simulink model "Parallel_n25_D2"  (R2012b)
settings: Solver=VariableStepDiscrete  StartTime=0.0  StopTime=TotalIterations  RelTol=1e-3
values from neighbouring files (symbols this model uses):
  bp = 12    [ConfigValidate.m]
  bpSNMemory = bp    (= 12)    [ConfigValidate.m]
  IterationsOrdering = 4000    [ConfigValidate.m]
  MaxCoordDistance = (abs(max(wx) - min(wx))+abs(max(wy) - min(wy)))^2    [ConfigValidate.m]
  N_limit = 0.01    [ConfigValidate.m]
  nBits = 9    [ConfigValidate.m]
  nBitsNSmemories = (ceil(log2(TotalIterations)))    [ConfigValidate.m]
  S_limit = 1    [ConfigValidate.m]
  SourceNodes = 2000    [ConfigValidate.m]
  ts = 1    [ConfigValidate.m]
  w1 = rand(1,Neurons)    [ConfigValidate.m]
  w2 = rand(1,Neurons)    [ConfigValidate.m]
  wx = zeros(1,Neurons)    [ConfigValidate.m]
  wy = zeros(1,Neurons)    [ConfigValidate.m]
  x1 = rand(SourceNodes,1)    [ConfigValidate.m]
  x2 = rand(SourceNodes,1)    [ConfigValidate.m]
libraries: xbsIndex_r4 x1652, dspsrcs4 x2, dspstat3 x2
(part 2 of 9)

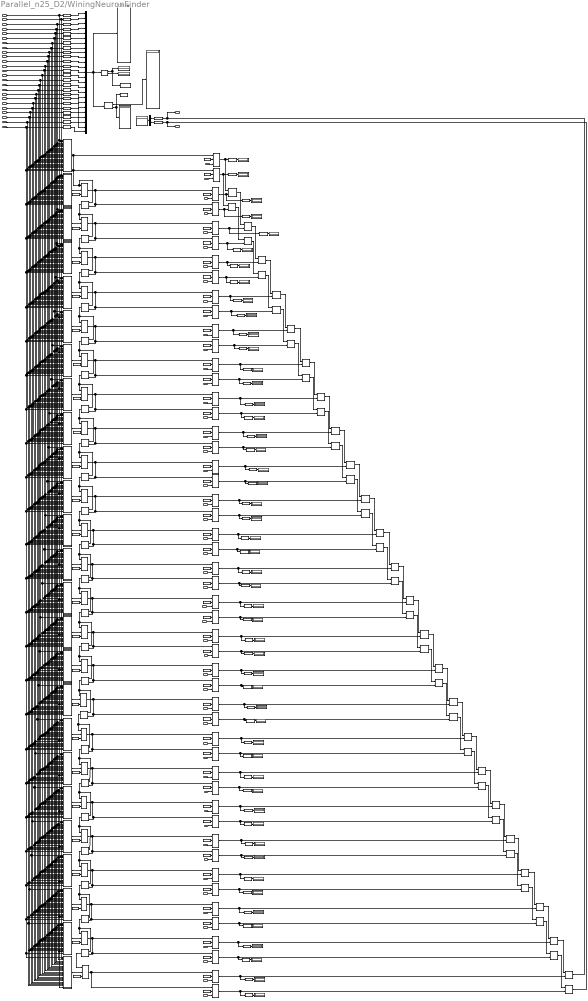
== system Parallel_n25_D2/WiningNeuronFinder ==
  dist_k1 : Inport
  dist_k2 : Inport  Port=2
  dist_k3 : Inport  Port=3
  dist_k4 : Inport  Port=4
  dist_k5 : Inport  Port=5
  dist_k6 : Inport  Port=6
  dist_k7 : Inport  Port=7
  dist_k8 : Inport  Port=8
  dist_k9 : Inport  Port=9
  dist_k10 : Inport  Port=10
  dist_k11 : Inport  Port=11
  dist_k12 : Inport  Port=12
  dist_k13 : Inport  Port=13
  dist_k14 : Inport  Port=14
  dist_k15 : Inport  Port=15
  dist_k16 : Inport  Port=16
  dist_k17 : Inport  Port=17
  dist_k18 : Inport  Port=18
  dist_k19 : Inport  Port=19
  dist_k20 : Inport  Port=20
  dist_k21 : Inport  Port=21
  dist_k22 : Inport  Port=22
  dist_k23 : Inport  Port=23
  dist_k24 : Inport  Port=24
  dist_k25 : Inport  Port=25
  wx_1 : Inport  Port=26
  wy_1 : Inport  Port=27
  wx_2 : Inport  Port=28
  wy_2 : Inport  Port=29
  wx_3 : Inport  Port=30
  wy_3 : Inport  Port=31
  wx_4 : Inport  Port=32
  wy_4 : Inport  Port=33
  wx_5 : Inport  Port=34
  wy_5 : Inport  Port=35
  wx_6 : Inport  Port=36
  wy_6 : Inport  Port=37
  wx_7 : Inport  Port=38
  wy_7 : Inport  Port=39
  wx_8 : Inport  Port=40
  wy_8 : Inport  Port=41
  wx_9 : Inport  Port=42
  wy_9 : Inport  Port=43
  wx_10 : Inport  Port=44
  wy_10 : Inport  Port=45
  wx_11 : Inport  Port=46
  wy_11 : Inport  Port=47
  wx_12 : Inport  Port=48
  wy_12 : Inport  Port=49
  wx_13 : Inport  Port=50
  wy_13 : Inport  Port=51
  wx_14 : Inport  Port=52
  wy_14 : Inport  Port=53
  wx_15 : Inport  Port=54
  wy_15 : Inport  Port=55
  wx_16 : Inport  Port=56
  wy_16 : Inport  Port=57
  wx_17 : Inport  Port=58
  wy_17 : Inport  Port=59
  wx_18 : Inport  Port=60
  wy_18 : Inport  Port=61
  wx_19 : Inport  Port=62
  wy_19 : Inport  Port=63
  wx_20 : Inport  Port=64
  wy_20 : Inport  Port=65
  wx_21 : Inport  Port=66
  wy_21 : Inport  Port=67
  wx_22 : Inport  Port=68
  wy_22 : Inport  Port=69
  wx_23 : Inport  Port=70
  wy_23 : Inport  Port=71
  wx_24 : Inport  Port=72
  wy_24 : Inport  Port=73
  wx_25 : Inport  Port=74
  wy_25 : Inport  Port=75
  Display{,1..55} (56 alike) : Display
  Gateway Out{,1..24,27..78} (77 alike) : xbsIndex_r4/Gateway Out  inherit_from_input=off  hdl_port=off  timing_constraint=None  locs_specified=off  LOCs={}  UseAsDAC=off  DACChannel='1'  block_type=gatewayout
  Logical{,1..22} (23 alike) : xbsIndex_r4/Logical  logical_function=OR  inputs=2  en=off  latency=0  precision=Full  arith_type=Unsigned  n_bits=16  bin_pt=0  align_bp=on  dbl_ovrd=off  block_type=logical
  LowerDist_n1 : Subsystem
  LowerDist_n10 : Subsystem
  LowerDist_n11 : Subsystem
  LowerDist_n12 : Subsystem
  LowerDist_n13 : Subsystem
  LowerDist_n14 : Subsystem
  LowerDist_n15 : Subsystem
  LowerDist_n16 : Subsystem
  LowerDist_n17 : Subsystem
  LowerDist_n18 : Subsystem
  LowerDist_n19 : Subsystem
  LowerDist_n2 : Subsystem
  LowerDist_n20 : Subsystem
  LowerDist_n21 : Subsystem
  LowerDist_n22 : Subsystem
  LowerDist_n23 : Subsystem
  LowerDist_n24 : Subsystem
  LowerDist_n25 : Subsystem
  LowerDist_n3 : Subsystem
  LowerDist_n4 : Subsystem
  LowerDist_n5 : Subsystem
  LowerDist_n6 : Subsystem
  LowerDist_n7 : Subsystem
  LowerDist_n8 : Subsystem
  LowerDist_n9 : Subsystem
  Minimum : dspstat3/Minimum  fcn=Value and Index  reset=None  InputProcessing=Columns as channels (frame based)  indexBase=One  operateOver=Each column  Dimension=1  colComp=on  operation=minimum  roiEnable=off  roiType=Rectangles  roiPortion=Entire ROI  roiOutput=Individual statistics for each ROI  roiFlag=off  roundingMode=Floor  overflowMode=off
  Mux : Mux  Inputs=25
  Mux2 : Mux  Inputs=2
  Sort : dspstat3/Sort  otype=Value and Index  dir=Ascending  sortAlg=Quick sort  accumDataTypeStr=Inherit: Same as product output  accumLastDataTypeStr=Inherit: Same as product output  roundingMode=Floor  overflowMode=off
  Sum_wxWinning_n{1..48} (48 alike) : xbsIndex_r4/AddSub  mode=Addition  use_carryin=off  use_carryout=off  en=off  latency=dAdd_CooperatingProcess  precision=User Defined  arith_type=Unsigned  n_bits=nbCoord  bin_pt=bpCoord  quantization=Truncate  overflow=Wrap  dbl_ovrd=off  use_behavioral_HDL=off  hw_selection=Fabric  pipelined=off  block_type=addsub
  To Workspace : ToWorkspace  VariableName=win_histH  SampleTime=ts
  To Workspace1 : ToWorkspace  VariableName=win_distH  SampleTime=ts
  wy_doMenor{,1..73} (74 alike) : xbsIndex_r4/Mux  inputs=2  en=off  latency=dMUX_CompetitiveProcess  precision=Full  arith_type=Unsigned  n_bits=16  bin_pt=14  quantization=Truncate  overflow=Wrap  dbl_ovrd=off  block_type=mux
  zero{,1..49} (50 alike) : xbsIndex_r4/Constant  const=0  gui_display_data_type=Fixed-point  arith_type=Unsigned  n_bits=nbCoord  bin_pt=bpCoord  preci_type=Single  exp_width=8  frac_width=24  explicit_period=on  period=ts  equ=P=C  opselect=C  inp2=PCIN>>17  opr=+  inp1=P  carry=CIN  dbl_ovrd=off  block_type=constant
  zero{50..73} (24 alike) : xbsIndex_r4/Constant  const=0  gui_display_data_type=Boolean  arith_type=Boolean  n_bits=nbCoord  bin_pt=bpCoord  preci_type=Single  exp_width=8  frac_width=24  explicit_period=on  period=ts  equ=P=C  opselect=C  inp2=PCIN>>17  opr=+  inp1=P  carry=CIN  dbl_ovrd=off  block_type=constant
  WinningNeuron_wx : Outport
  WinningNeuron_wy : Outport  Port=2
  wires:
  dist_k6/1 -> LowerDist_n25/6(In6), LowerDist_n24/6(In6), LowerDist_n23/6(In6), LowerDist_n22/6(In6), LowerDist_n21/6(In6), LowerDist_n20/6(In6), LowerDist_n19/6(In6), LowerDist_n18/6(In6), LowerDist_n17/6(In6), LowerDist_n16/6(In6), LowerDist_n15/6(In6), LowerDist_n14/6(In6), LowerDist_n13/6(In6), LowerDist_n12/6(In6), LowerDist_n11/6(In6), LowerDist_n10/6(In6), LowerDist_n9/6(In6), LowerDist_n8/6(In6), LowerDist_n7/6(In6), LowerDist_n6/1(In1), LowerDist_n5/6(In6), LowerDist_n4/6(In6), LowerDist_n3/6(In6), LowerDist_n2/6(In6), LowerDist_n1/6(In6), Gateway Out5/1
  wy_1/1 -> wy_doMenor1/3
  wx_2/1 -> wy_doMenor2/3
  wy_2/1 -> wy_doMenor3/3
  wx_3/1 -> wy_doMenor4/3
  wy_3/1 -> wy_doMenor5/3
  wx_4/1 -> wy_doMenor6/3
  wy_4/1 -> wy_doMenor7/3
  wx_5/1 -> wy_doMenor8/3
  wy_5/1 -> wy_doMenor9/3
  wx_6/1 -> wy_doMenor10/3
  wy_6/1 -> wy_doMenor11/3
  wx_7/1 -> wy_doMenor12/3
  wy_7/1 -> wy_doMenor13/3
  wx_8/1 -> wy_doMenor14/3
  wy_8/1 -> wy_doMenor15/3
  wx_9/1 -> wy_doMenor16/3
  wy_9/1 -> wy_doMenor17/3
  wx_10/1 -> wy_doMenor18/3
  wy_10/1 -> wy_doMenor19/3
  wx_11/1 -> wy_doMenor20/3
  wy_11/1 -> wy_doMenor21/3
  wx_12/1 -> wy_doMenor22/3
  wy_12/1 -> wy_doMenor23/3
  wx_13/1 -> wy_doMenor24/3
  wy_13/1 -> wy_doMenor25/3
  wx_14/1 -> wy_doMenor26/3
  wy_14/1 -> wy_doMenor27/3
  wx_15/1 -> wy_doMenor28/3
  wy_15/1 -> wy_doMenor29/3
  wx_16/1 -> wy_doMenor30/3
  wy_16/1 -> wy_doMenor31/3
  wx_17/1 -> wy_doMenor32/3
  wy_17/1 -> wy_doMenor33/3
  wx_18/1 -> wy_doMenor34/3
  wy_18/1 -> wy_doMenor35/3
  wx_19/1 -> wy_doMenor36/3
  wy_19/1 -> wy_doMenor37/3
  wx_20/1 -> wy_doMenor38/3
  wy_20/1 -> wy_doMenor39/3
  wx_21/1 -> wy_doMenor40/3
  wy_21/1 -> wy_doMenor41/3
  wx_22/1 -> wy_doMenor42/3
  wy_22/1 -> wy_doMenor43/3
  wx_23/1 -> wy_doMenor44/3
  wy_23/1 -> wy_doMenor45/3
  wx_24/1 -> wy_doMenor46/3
  wy_24/1 -> wy_doMenor47/3
  wx_25/1 -> wy_doMenor48/3
  wy_25/1 -> wy_doMenor49/3
  wx_1/1 -> wy_doMenor/3
  Gateway Out6/1 -> Mux/7
  Gateway Out5/1 -> Mux/6
  Gateway Out7/1 -> Mux/8
  Gateway Out4/1 -> Mux/5
  Gateway Out8/1 -> Mux/9
  Gateway Out1/1 -> Mux/2
  Gateway Out3/1 -> Mux/4
  Gateway Out2/1 -> Mux/3
  Gateway Out10/1 -> Mux/11
  Gateway Out11/1 -> Mux/12
  Gateway Out9/1 -> Mux/10
  Gateway Out/1 -> Mux/1
  Gateway Out12/1 -> Mux/13
  Gateway Out22/1 -> Mux/17
  Gateway Out13/1 -> Mux/14
  Gateway Out14/1 -> Mux/15
  Gateway Out15/1 -> Mux/16
  Gateway Out23/1 -> Mux/18
  Gateway Out16/1 -> Mux/20
  Gateway Out17/1 -> Mux/21
  Gateway Out24/1 -> Mux/19
  Gateway Out18/1 -> Mux/22
  Gateway Out20/1 -> Mux/24
  Gateway Out21/1 -> Mux/25
  Gateway Out19/1 -> Mux/23
  dist_k3/1 -> LowerDist_n1/3(In3), LowerDist_n25/3(In3), LowerDist_n24/3(In3), LowerDist_n23/3(In3), LowerDist_n22/3(In3), LowerDist_n21/3(In3), LowerDist_n20/3(In3), LowerDist_n19/3(In3), LowerDist_n18/3(In3), LowerDist_n17/3(In3), LowerDist_n16/3(In3), LowerDist_n15/3(In3), LowerDist_n14/3(In3), LowerDist_n13/3(In3), LowerDist_n12/3(In3), LowerDist_n11/3(In3), LowerDist_n10/3(In3), LowerDist_n9/3(In3), LowerDist_n8/3(In3), LowerDist_n7/3(In3), LowerDist_n6/3(In3), LowerDist_n5/3(In3), LowerDist_n4/3(In3), LowerDist_n3/1(In1), LowerDist_n2/3(In3), Gateway Out2/1
  dist_k25/1 -> LowerDist_n6/25(In25), LowerDist_n12/25(In25), LowerDist_n15/25(In25), LowerDist_n21/25(In25), LowerDist_n25/1(In1), LowerDist_n24/25(In25), LowerDist_n23/25(In25), LowerDist_n22/25(In25), LowerDist_n20/25(In25), LowerDist_n19/25(In25), LowerDist_n18/25(In25), LowerDist_n17/25(In25), LowerDist_n16/25(In25), LowerDist_n14/25(In25), LowerDist_n13/25(In25), LowerDist_n11/25(In25), LowerDist_n10/25(In25), LowerDist_n9/25(In25), LowerDist_n8/25(In25), LowerDist_n7/25(In25), LowerDist_n5/25(In25), LowerDist_n4/25(In25), LowerDist_n3/25(In25), LowerDist_n2/25(In25), LowerDist_n1/25(In25), Gateway Out21/1
  dist_k15/1 -> LowerDist_n20/15(In15), LowerDist_n25/15(In15), LowerDist_n24/15(In15), LowerDist_n23/15(In15), LowerDist_n22/15(In15), LowerDist_n21/15(In15), LowerDist_n19/15(In15), LowerDist_n18/15(In15), LowerDist_n17/15(In15), LowerDist_n16/15(In15), LowerDist_n15/1(In1), LowerDist_n14/15(In15), LowerDist_n13/15(In15), LowerDist_n12/15(In15), LowerDist_n11/15(In15), LowerDist_n10/15(In15), LowerDist_n9/15(In15), LowerDist_n8/15(In15), LowerDist_n7/15(In15), LowerDist_n6/15(In15), LowerDist_n5/15(In15), LowerDist_n4/15(In15), LowerDist_n3/15(In15), LowerDist_n2/15(In15), LowerDist_n1/15(In15), Gateway Out14/1
  dist_k2/1 -> LowerDist_n25/2(In2), LowerDist_n24/2(In2), LowerDist_n23/2(In2), LowerDist_n22/2(In2), LowerDist_n21/2(In2), LowerDist_n20/2(In2), LowerDist_n19/2(In2), LowerDist_n18/2(In2), LowerDist_n17/2(In2), LowerDist_n16/2(In2), LowerDist_n15/2(In2), LowerDist_n14/2(In2), LowerDist_n13/2(In2), LowerDist_n12/2(In2), LowerDist_n11/2(In2), LowerDist_n10/2(In2), LowerDist_n9/2(In2), LowerDist_n8/2(In2), LowerDist_n7/2(In2), LowerDist_n6/2(In2), LowerDist_n5/2(In2), LowerDist_n4/2(In2), LowerDist_n3/2(In2), LowerDist_n2/1(In1), LowerDist_n1/2(In2), Gateway Out1/1
  dist_k4/1 -> LowerDist_n2/4(In4), LowerDist_n8/4(In4), LowerDist_n25/4(In4), LowerDist_n24/4(In4), LowerDist_n23/4(In4), LowerDist_n22/4(In4), LowerDist_n21/4(In4), LowerDist_n20/4(In4), LowerDist_n19/4(In4), LowerDist_n18/4(In4), LowerDist_n17/4(In4), LowerDist_n16/4(In4), LowerDist_n15/4(In4), LowerDist_n14/4(In4), LowerDist_n13/4(In4), LowerDist_n12/4(In4), LowerDist_n11/4(In4), LowerDist_n10/4(In4), LowerDist_n9/4(In4), LowerDist_n7/4(In4), LowerDist_n6/4(In4), LowerDist_n5/4(In4), LowerDist_n4/1(In1), LowerDist_n3/4(In4), LowerDist_n1/4(In4), Gateway Out3/1
  dist_k7/1 -> LowerDist_n25/7(In7), LowerDist_n24/7(In7), LowerDist_n23/7(In7), LowerDist_n22/7(In7), LowerDist_n21/7(In7), LowerDist_n20/7(In7), LowerDist_n19/7(In7), LowerDist_n18/7(In7), LowerDist_n17/7(In7), LowerDist_n16/7(In7), LowerDist_n15/7(In7), LowerDist_n14/7(In7), LowerDist_n13/7(In7), LowerDist_n12/7(In7), LowerDist_n11/7(In7), LowerDist_n10/7(In7), LowerDist_n9/7(In7), LowerDist_n8/7(In7), LowerDist_n7/1(In1), LowerDist_n6/7(In7), LowerDist_n5/7(In7), LowerDist_n4/7(In7), LowerDist_n3/7(In7), LowerDist_n2/7(In7), LowerDist_n1/7(In7), Gateway Out6/1
  dist_k8/1 -> LowerDist_n8/1(In1), LowerDist_n25/8(In8), LowerDist_n24/8(In8), LowerDist_n23/8(In8), LowerDist_n22/8(In8), LowerDist_n21/8(In8), LowerDist_n20/8(In8), LowerDist_n19/8(In8), LowerDist_n18/8(In8), LowerDist_n17/8(In8), LowerDist_n16/8(In8), LowerDist_n15/8(In8), LowerDist_n14/8(In8), LowerDist_n13/8(In8), LowerDist_n12/8(In8), LowerDist_n11/8(In8), LowerDist_n10/8(In8), LowerDist_n9/8(In8), LowerDist_n7/8(In8), LowerDist_n6/8(In8), LowerDist_n5/8(In8), LowerDist_n4/8(In8), LowerDist_n3/8(In8), LowerDist_n2/8(In8), LowerDist_n1/8(In8), Gateway Out7/1
  dist_k9/1 -> LowerDist_n20/9(In9), LowerDist_n22/9(In9), LowerDist_n24/9(In9), LowerDist_n25/9(In9), LowerDist_n23/9(In9), LowerDist_n21/9(In9), LowerDist_n19/9(In9), LowerDist_n18/9(In9), LowerDist_n17/9(In9), LowerDist_n16/9(In9), LowerDist_n15/9(In9), LowerDist_n14/9(In9), LowerDist_n13/9(In9), LowerDist_n12/9(In9), LowerDist_n11/9(In9), LowerDist_n10/9(In9), LowerDist_n9/1(In1), LowerDist_n8/9(In9), LowerDist_n7/9(In9), LowerDist_n6/9(In9), LowerDist_n5/9(In9), LowerDist_n4/9(In9), LowerDist_n3/9(In9), LowerDist_n2/9(In9), LowerDist_n1/9(In9), Gateway Out8/1
  dist_k10/1 -> LowerDist_n9/10(In10), LowerDist_n25/10(In10), LowerDist_n24/10(In10), LowerDist_n23/10(In10), LowerDist_n22/10(In10), LowerDist_n21/10(In10), LowerDist_n20/10(In10), LowerDist_n19/10(In10), LowerDist_n18/10(In10), LowerDist_n17/10(In10), LowerDist_n16/10(In10), LowerDist_n15/10(In10), LowerDist_n14/10(In10), LowerDist_n13/10(In10), LowerDist_n12/10(In10), LowerDist_n11/10(In10), LowerDist_n10/1(In1), LowerDist_n8/10(In10), LowerDist_n7/10(In10), LowerDist_n6/10(In10), LowerDist_n5/10(In10), LowerDist_n4/10(In10), LowerDist_n3/10(In10), LowerDist_n2/10(In10), LowerDist_n1/10(In10), Gateway Out9/1
  dist_k11/1 -> LowerDist_n11/1(In1), LowerDist_n25/11(In11), LowerDist_n24/11(In11), LowerDist_n23/11(In11), LowerDist_n22/11(In11), LowerDist_n21/11(In11), LowerDist_n20/11(In11), LowerDist_n19/11(In11), LowerDist_n18/11(In11), LowerDist_n17/11(In11), LowerDist_n16/11(In11), LowerDist_n15/11(In11), LowerDist_n14/11(In11), LowerDist_n13/11(In11), LowerDist_n12/11(In11), LowerDist_n10/11(In11), LowerDist_n9/11(In11), LowerDist_n8/11(In11), LowerDist_n7/11(In11), LowerDist_n6/11(In11), LowerDist_n5/11(In11), LowerDist_n4/11(In11), LowerDist_n3/11(In11), LowerDist_n2/11(In11), LowerDist_n1/11(In11), Gateway Out10/1
  dist_k12/1 -> LowerDist_n11/12(In12), LowerDist_n23/12(In12), LowerDist_n25/12(In12), LowerDist_n24/12(In12), LowerDist_n22/12(In12), LowerDist_n21/12(In12), LowerDist_n20/12(In12), LowerDist_n19/12(In12), LowerDist_n18/12(In12), LowerDist_n17/12(In12), LowerDist_n16/12(In12), LowerDist_n15/12(In12), LowerDist_n14/12(In12), LowerDist_n13/12(In12), LowerDist_n12/1(In1), LowerDist_n10/12(In12), LowerDist_n9/12(In12), LowerDist_n8/12(In12), LowerDist_n7/12(In12), LowerDist_n6/12(In12), LowerDist_n5/12(In12), LowerDist_n4/12(In12), LowerDist_n3/12(In12), LowerDist_n2/12(In12), LowerDist_n1/12(In12), Gateway Out11/1
  dist_k13/1 -> LowerDist_n12/13(In13), LowerDist_n25/13(In13), LowerDist_n24/13(In13), LowerDist_n23/13(In13), LowerDist_n22/13(In13), LowerDist_n21/13(In13), LowerDist_n20/13(In13), LowerDist_n19/13(In13), LowerDist_n18/13(In13), LowerDist_n17/13(In13), LowerDist_n16/13(In13), LowerDist_n15/13(In13), LowerDist_n14/13(In13), LowerDist_n13/1(In1), LowerDist_n11/13(In13), LowerDist_n10/13(In13), LowerDist_n9/13(In13), LowerDist_n8/13(In13), LowerDist_n7/13(In13), LowerDist_n6/13(In13), LowerDist_n5/13(In13), LowerDist_n4/13(In13), LowerDist_n3/13(In13), LowerDist_n2/13(In13), LowerDist_n1/13(In13), Gateway Out12/1
  dist_k14/1 -> LowerDist_n14/1(In1), LowerDist_n21/14(In14), LowerDist_n25/14(In14), LowerDist_n24/14(In14), LowerDist_n23/14(In14), LowerDist_n22/14(In14), LowerDist_n20/14(In14), LowerDist_n19/14(In14), LowerDist_n18/14(In14), LowerDist_n17/14(In14), LowerDist_n16/14(In14), LowerDist_n15/14(In14), LowerDist_n13/14(In14), LowerDist_n12/14(In14), LowerDist_n11/14(In14), LowerDist_n10/14(In14), LowerDist_n9/14(In14), LowerDist_n8/14(In14), LowerDist_n7/14(In14), LowerDist_n6/14(In14), LowerDist_n5/14(In14), LowerDist_n4/14(In14), LowerDist_n3/14(In14), LowerDist_n2/14(In14), LowerDist_n1/14(In14), Gateway Out13/1
  dist_k16/1 -> LowerDist_n1/16(In16), LowerDist_n10/16(In16), LowerDist_n15/16(In16), LowerDist_n25/16(In16), LowerDist_n24/16(In16), LowerDist_n23/16(In16), LowerDist_n22/16(In16), LowerDist_n21/16(In16), LowerDist_n20/16(In16), LowerDist_n19/16(In16), LowerDist_n18/16(In16), LowerDist_n17/16(In16), LowerDist_n16/1(In1), LowerDist_n14/16(In16), LowerDist_n13/16(In16), LowerDist_n12/16(In16), LowerDist_n11/16(In16), LowerDist_n9/16(In16), LowerDist_n8/16(In16), LowerDist_n7/16(In16), LowerDist_n6/16(In16), LowerDist_n5/16(In16), LowerDist_n4/16(In16), LowerDist_n3/16(In16), LowerDist_n2/16(In16), Gateway Out15/1
  dist_k17/1 -> LowerDist_n1/17(In17), LowerDist_n13/17(In17), LowerDist_n25/17(In17), LowerDist_n24/17(In17), LowerDist_n23/17(In17), LowerDist_n22/17(In17), LowerDist_n21/17(In17), LowerDist_n20/17(In17), LowerDist_n19/17(In17), LowerDist_n18/17(In17), LowerDist_n17/1(In1), LowerDist_n16/17(In17), LowerDist_n15/17(In17), LowerDist_n14/17(In17), LowerDist_n12/17(In17), LowerDist_n11/17(In17), LowerDist_n10/17(In17), LowerDist_n9/17(In17), LowerDist_n8/17(In17), LowerDist_n7/17(In17), LowerDist_n6/17(In17), LowerDist_n5/17(In17), LowerDist_n4/17(In17), LowerDist_n3/17(In17), LowerDist_n2/17(In17), Gateway Out22/1
  dist_k18/1 -> LowerDist_n17/18(In18), LowerDist_n25/18(In18), LowerDist_n24/18(In18), LowerDist_n23/18(In18), LowerDist_n22/18(In18), LowerDist_n21/18(In18), LowerDist_n20/18(In18), LowerDist_n19/18(In18), LowerDist_n18/1(In1), LowerDist_n16/18(In18), LowerDist_n15/18(In18), LowerDist_n14/18(In18), LowerDist_n13/18(In18), LowerDist_n12/18(In18), LowerDist_n11/18(In18), LowerDist_n10/18(In18), LowerDist_n9/18(In18), LowerDist_n8/18(In18), LowerDist_n7/18(In18), LowerDist_n6/18(In18), LowerDist_n5/18(In18), LowerDist_n4/18(In18), LowerDist_n3/18(In18), LowerDist_n2/18(In18), LowerDist_n1/18(In18), Gateway Out23/1
  dist_k19/1 -> LowerDist_n25/19(In19), LowerDist_n24/19(In19), LowerDist_n23/19(In19), LowerDist_n22/19(In19), LowerDist_n21/19(In19), LowerDist_n20/19(In19), LowerDist_n19/1(In1), LowerDist_n18/19(In19), LowerDist_n17/19(In19), LowerDist_n16/19(In19), LowerDist_n15/19(In19), LowerDist_n14/19(In19), LowerDist_n13/19(In19), LowerDist_n12/19(In19), LowerDist_n11/19(In19), LowerDist_n10/19(In19), LowerDist_n9/19(In19), LowerDist_n8/19(In19), LowerDist_n7/19(In19), LowerDist_n6/19(In19), LowerDist_n5/19(In19), LowerDist_n4/19(In19), LowerDist_n3/19(In19), LowerDist_n2/19(In19), LowerDist_n1/19(In19), Gateway Out24/1
  dist_k21/1 -> LowerDist_n9/21(In21), LowerDist_n25/21(In21), LowerDist_n24/21(In21), LowerDist_n23/21(In21), LowerDist_n22/21(In21), LowerDist_n21/1(In1), LowerDist_n20/21(In21), LowerDist_n19/21(In21), LowerDist_n18/21(In21), LowerDist_n17/21(In21), LowerDist_n16/21(In21), LowerDist_n15/21(In21), LowerDist_n14/21(In21), LowerDist_n13/21(In21), LowerDist_n12/21(In21), LowerDist_n11/21(In21), LowerDist_n10/21(In21), LowerDist_n8/21(In21), LowerDist_n7/21(In21), LowerDist_n6/21(In21), LowerDist_n5/21(In21), LowerDist_n4/21(In21), LowerDist_n3/21(In21), LowerDist_n2/21(In21), LowerDist_n1/21(In21), Gateway Out17/1
  dist_k22/1 -> LowerDist_n7/22(In22), LowerDist_n25/22(In22), LowerDist_n24/22(In22), LowerDist_n23/22(In22), LowerDist_n22/1(In1), LowerDist_n21/22(In22), LowerDist_n20/22(In22), LowerDist_n19/22(In22), LowerDist_n18/22(In22), LowerDist_n17/22(In22), LowerDist_n16/22(In22), LowerDist_n15/22(In22), LowerDist_n14/22(In22), LowerDist_n13/22(In22), LowerDist_n12/22(In22), LowerDist_n11/22(In22), LowerDist_n10/22(In22), LowerDist_n9/22(In22), LowerDist_n8/22(In22), LowerDist_n6/22(In22), LowerDist_n5/22(In22), LowerDist_n4/22(In22), LowerDist_n3/22(In22), LowerDist_n2/22(In22), LowerDist_n1/22(In22), Gateway Out18/1
  dist_k23/1 -> LowerDist_n25/23(In23), LowerDist_n24/23(In23), LowerDist_n23/1(In1), LowerDist_n22/23(In23), LowerDist_n21/23(In23), LowerDist_n20/23(In23), LowerDist_n19/23(In23), LowerDist_n18/23(In23), LowerDist_n17/23(In23), LowerDist_n16/23(In23), LowerDist_n15/23(In23), LowerDist_n14/23(In23), LowerDist_n13/23(In23), LowerDist_n12/23(In23), LowerDist_n11/23(In23), LowerDist_n10/23(In23), LowerDist_n9/23(In23), LowerDist_n8/23(In23), LowerDist_n7/23(In23), LowerDist_n6/23(In23), LowerDist_n5/23(In23), LowerDist_n4/23(In23), LowerDist_n3/23(In23), LowerDist_n2/23(In23), LowerDist_n1/23(In23), Gateway Out19/1
  dist_k24/1 -> LowerDist_n25/24(In24), LowerDist_n24/1(In1), LowerDist_n23/24(In24), LowerDist_n22/24(In24), LowerDist_n21/24(In24), LowerDist_n20/24(In24), LowerDist_n19/24(In24), LowerDist_n18/24(In24), LowerDist_n17/24(In24), LowerDist_n16/24(In24), LowerDist_n15/24(In24), LowerDist_n14/24(In24), LowerDist_n13/24(In24), LowerDist_n12/24(In24), LowerDist_n11/24(In24), LowerDist_n10/24(In24), LowerDist_n9/24(In24), LowerDist_n8/24(In24), LowerDist_n7/24(In24), LowerDist_n6/24(In24), LowerDist_n5/24(In24), LowerDist_n4/24(In24), LowerDist_n3/24(In24), LowerDist_n2/24(In24), LowerDist_n1/24(In24), Gateway Out20/1
  dist_k1/1 -> LowerDist_n1/1(In1), LowerDist_n4/4(In4), LowerDist_n25/25(In25), LowerDist_n24/24(In24), LowerDist_n23/23(In23), LowerDist_n22/22(In22), LowerDist_n21/21(In21), LowerDist_n20/20(In20), LowerDist_n19/19(In19), LowerDist_n18/18(In18), LowerDist_n17/17(In17), LowerDist_n16/16(In16), LowerDist_n15/15(In15), LowerDist_n14/14(In14), LowerDist_n13/13(In13), LowerDist_n12/12(In12), LowerDist_n11/11(In11), LowerDist_n10/10(In10), LowerDist_n9/9(In9), LowerDist_n8/8(In8), LowerDist_n7/7(In7), LowerDist_n6/6(In6), LowerDist_n5/5(In5), LowerDist_n3/3(In3), LowerDist_n2/2(In2), Gateway Out/1
  dist_k20/1 -> LowerDist_n14/20(In20), LowerDist_n25/20(In20), LowerDist_n24/20(In20), LowerDist_n23/20(In20), LowerDist_n22/20(In20), LowerDist_n21/20(In20), LowerDist_n20/1(In1), LowerDist_n19/20(In20), LowerDist_n18/20(In20), LowerDist_n17/20(In20), LowerDist_n16/20(In20), LowerDist_n15/20(In20), LowerDist_n13/20(In20), LowerDist_n12/20(In20), LowerDist_n11/20(In20), LowerDist_n10/20(In20), LowerDist_n9/20(In20), LowerDist_n8/20(In20), LowerDist_n7/20(In20), LowerDist_n6/20(In20), LowerDist_n5/20(In20), LowerDist_n4/20(In20), LowerDist_n3/20(In20), LowerDist_n2/20(In20), LowerDist_n1/20(In20), Gateway Out16/1
  zero/1 -> wy_doMenor/2
  zero1/1 -> wy_doMenor1/2
  zero2/1 -> wy_doMenor2/2
  zero3/1 -> wy_doMenor3/2
  zero4/1 -> wy_doMenor4/2
  zero5/1 -> wy_doMenor5/2
  zero6/1 -> wy_doMenor6/2
  zero7/1 -> wy_doMenor7/2
  zero8/1 -> wy_doMenor8/2
  zero9/1 -> wy_doMenor9/2
  zero10/1 -> wy_doMenor10/2
  zero11/1 -> wy_doMenor11/2
  zero12/1 -> wy_doMenor12/2
  zero13/1 -> wy_doMenor13/2
  zero14/1 -> wy_doMenor14/2
  zero15/1 -> wy_doMenor15/2
  zero16/1 -> wy_doMenor16/2
  zero17/1 -> wy_doMenor17/2
  zero18/1 -> wy_doMenor18/2
  zero19/1 -> wy_doMenor19/2
  zero20/1 -> wy_doMenor20/2
  zero21/1 -> wy_doMenor21/2
  zero22/1 -> wy_doMenor22/2
  zero23/1 -> wy_doMenor23/2
  zero24/1 -> wy_doMenor24/2
  zero25/1 -> wy_doMenor25/2
  zero26/1 -> wy_doMenor26/2
  zero27/1 -> wy_doMenor27/2
  zero28/1 -> wy_doMenor28/2
  zero29/1 -> wy_doMenor29/2
  zero30/1 -> wy_doMenor30/2
  zero31/1 -> wy_doMenor31/2
  zero32/1 -> wy_doMenor32/2
  zero33/1 -> wy_doMenor33/2
  zero34/1 -> wy_doMenor34/2
  zero35/1 -> wy_doMenor35/2
  zero36/1 -> wy_doMenor36/2
  zero37/1 -> wy_doMenor37/2
  zero38/1 -> wy_doMenor38/2
  zero39/1 -> wy_doMenor39/2
  zero40/1 -> wy_doMenor40/2
  zero41/1 -> wy_doMenor41/2
  zero42/1 -> wy_doMenor42/2
  zero43/1 -> wy_doMenor43/2
  zero44/1 -> wy_doMenor44/2
  zero45/1 -> wy_doMenor45/2
  zero46/1 -> wy_doMenor46/2
  zero47/1 -> wy_doMenor47/2
  zero48/1 -> wy_doMenor48/2
  zero49/1 -> wy_doMenor49/2
  wy_doMenor/1 -> Gateway Out29/1, Sum_wxWinning_n1/1
  wy_doMenor2/1 -> Gateway Out31/1, Sum_wxWinning_n1/2
  wy_doMenor1/1 -> Gateway Out30/1, Sum_wxWinning_n2/1
  wy_doMenor3/1 -> Gateway Out32/1, Sum_wxWinning_n2/2
  Sum_wxWinning_n1/1 -> Sum_wxWinning_n3/1
  Sum_wxWinning_n2/1 -> Sum_wxWinning_n4/1
  wy_doMenor4/1 -> Gateway Out34/1, Sum_wxWinning_n3/2
  wy_doMenor5/1 -> Gateway Out33/1, Sum_wxWinning_n4/2
  Sum_wxWinning_n3/1 -> Sum_wxWinning_n5/1
  Sum_wxWinning_n4/1 -> Sum_wxWinning_n6/1
  wy_doMenor6/1 -> Gateway Out35/1, Sum_wxWinning_n5/2
  wy_doMenor7/1 -> Gateway Out36/1, Sum_wxWinning_n6/2
  Sum_wxWinning_n5/1 -> Sum_wxWinning_n7/1
  Sum_wxWinning_n6/1 -> Sum_wxWinning_n8/1
  wy_doMenor9/1 -> Gateway Out38/1, Sum_wxWinning_n8/2
  Sum_wxWinning_n7/1 -> Sum_wxWinning_n9/1
  Sum_wxWinning_n8/1 -> Sum_wxWinning_n10/1
  wy_doMenor10/1 -> Gateway Out39/1, Sum_wxWinning_n9/2
  wy_doMenor11/1 -> Gateway Out40/1, Sum_wxWinning_n10/2
  Sum_wxWinning_n9/1 -> Sum_wxWinning_n12/1
  Sum_wxWinning_n10/1 -> Sum_wxWinning_n11/1
  wy_doMenor12/1 -> Gateway Out41/1, Sum_wxWinning_n12/2
  wy_doMenor13/1 -> Gateway Out42/1, Sum_wxWinning_n11/2
  Sum_wxWinning_n12/1 -> Sum_wxWinning_n14/1
  Sum_wxWinning_n11/1 -> Sum_wxWinning_n13/1
  wy_doMenor14/1 -> Gateway Out43/1, Sum_wxWinning_n14/2
  wy_doMenor15/1 -> Gateway Out44/1, Sum_wxWinning_n13/2
  Sum_wxWinning_n14/1 -> Sum_wxWinning_n16/1
  Sum_wxWinning_n13/1 -> Sum_wxWinning_n15/1
  wy_doMenor16/1 -> Gateway Out45/1, Sum_wxWinning_n16/2
  wy_doMenor17/1 -> Gateway Out46/1, Sum_wxWinning_n15/2
  Sum_wxWinning_n16/1 -> Sum_wxWinning_n18/1
  Sum_wxWinning_n15/1 -> Sum_wxWinning_n17/1
  wy_doMenor18/1 -> Gateway Out47/1, Sum_wxWinning_n18/2
  wy_doMenor19/1 -> Gateway Out48/1, Sum_wxWinning_n17/2
  Sum_wxWinning_n18/1 -> Sum_wxWinning_n20/1
  Sum_wxWinning_n17/1 -> Sum_wxWinning_n19/1
  wy_doMenor20/1 -> Gateway Out49/1, Sum_wxWinning_n20/2
  wy_doMenor21/1 -> Gateway Out50/1, Sum_wxWinning_n19/2
  Sum_wxWinning_n20/1 -> Sum_wxWinning_n22/1
  Sum_wxWinning_n19/1 -> Sum_wxWinning_n21/1
  wy_doMenor22/1 -> Gateway Out51/1, Sum_wxWinning_n22/2
  Sum_wxWinning_n22/1 -> Sum_wxWinning_n24/1
  Sum_wxWinning_n21/1 -> Sum_wxWinning_n23/1
  wy_doMenor24/1 -> Gateway Out53/1, Sum_wxWinning_n24/2
  wy_doMenor25/1 -> Gateway Out54/1, Sum_wxWinning_n23/2
  Sum_wxWinning_n24/1 -> Sum_wxWinning_n26/1
  Sum_wxWinning_n23/1 -> Sum_wxWinning_n25/1
  wy_doMenor26/1 -> Gateway Out55/1, Sum_wxWinning_n26/2
  wy_doMenor27/1 -> Gateway Out56/1, Sum_wxWinning_n25/2
  Sum_wxWinning_n26/1 -> Sum_wxWinning_n28/1
  Sum_wxWinning_n25/1 -> Sum_wxWinning_n27/1
  wy_doMenor28/1 -> Gateway Out57/1, Sum_wxWinning_n28/2
  wy_doMenor29/1 -> Gateway Out58/1, Sum_wxWinning_n27/2
  Sum_wxWinning_n28/1 -> Sum_wxWinning_n30/1
  Sum_wxWinning_n27/1 -> Sum_wxWinning_n29/1
  wy_doMenor30/1 -> Gateway Out59/1, Sum_wxWinning_n30/2
  wy_doMenor31/1 -> Gateway Out60/1, Sum_wxWinning_n29/2
  Sum_wxWinning_n30/1 -> Sum_wxWinning_n32/1
  Sum_wxWinning_n29/1 -> Sum_wxWinning_n31/1
  wy_doMenor32/1 -> Gateway Out61/1, Sum_wxWinning_n32/2
  wy_doMenor33/1 -> Gateway Out62/1, Sum_wxWinning_n31/2
  Sum_wxWinning_n32/1 -> Sum_wxWinning_n34/1
  Sum_wxWinning_n31/1 -> Sum_wxWinning_n33/1
  wy_doMenor34/1 -> Gateway Out63/1, Sum_wxWinning_n34/2
  wy_doMenor35/1 -> Gateway Out64/1, Sum_wxWinning_n33/2
  Sum_wxWinning_n34/1 -> Sum_wxWinning_n36/1
  Sum_wxWinning_n33/1 -> Sum_wxWinning_n35/1
  wy_doMenor36/1 -> Gateway Out65/1, Sum_wxWinning_n36/2
  wy_doMenor37/1 -> Gateway Out66/1, Sum_wxWinning_n35/2
  Sum_wxWinning_n36/1 -> Sum_wxWinning_n38/1
  Sum_wxWinning_n35/1 -> Sum_wxWinning_n37/1
  wy_doMenor38/1 -> Gateway Out67/1, Sum_wxWinning_n38/2
  wy_doMenor39/1 -> Gateway Out68/1, Sum_wxWinning_n37/2
  Sum_wxWinning_n38/1 -> Sum_wxWinning_n40/1
  Sum_wxWinning_n37/1 -> Sum_wxWinning_n39/1
  wy_doMenor40/1 -> Gateway Out69/1, Sum_wxWinning_n40/2
  wy_doMenor41/1 -> Gateway Out70/1, Sum_wxWinning_n39/2
  Sum_wxWinning_n40/1 -> Sum_wxWinning_n42/1
  Sum_wxWinning_n39/1 -> Sum_wxWinning_n41/1
  wy_doMenor42/1 -> Gateway Out71/1, Sum_wxWinning_n42/2
  wy_doMenor43/1 -> Gateway Out72/1, Sum_wxWinning_n41/2
  Sum_wxWinning_n42/1 -> Sum_wxWinning_n44/1
  Sum_wxWinning_n41/1 -> Sum_wxWinning_n43/1
  wy_doMenor44/1 -> Gateway Out73/1, Sum_wxWinning_n44/2
  Sum_wxWinning_n44/1 -> Sum_wxWinning_n46/1
  Sum_wxWinning_n43/1 -> Sum_wxWinning_n45/1
  wy_doMenor46/1 -> Gateway Out75/1, Sum_wxWinning_n46/2
  wy_doMenor47/1 -> Gateway Out76/1, Sum_wxWinning_n45/2
  Sum_wxWinning_n46/1 -> Sum_wxWinning_n48/1
  Sum_wxWinning_n45/1 -> Sum_wxWinning_n47/1
  wy_doMenor48/1 -> Gateway Out77/1, Sum_wxWinning_n48/2
  wy_doMenor49/1 -> Gateway Out78/1, Sum_wxWinning_n47/2
  Gateway Out28/1 -> Mux2/2
  Gateway Out27/1 -> Mux2/1
  Mux2/1 -> Display3/1
  Sum_wxWinning_n48/1 -> WinningNeuron_wx/1, Gateway Out27/1
  Sum_wxWinning_n47/1 -> WinningNeuron_wy/1, Gateway Out28/1
  Gateway Out29/1 -> Display4/1
  Gateway Out30/1 -> Display5/1
  Gateway Out31/1 -> Display6/1
  Gateway Out32/1 -> Display7/1
  Gateway Out33/1 -> Display8/1
  Gateway Out34/1 -> Display9/1
  Gateway Out35/1 -> Display10/1
  Gateway Out36/1 -> Display11/1
  Gateway Out37/1 -> Display12/1
  wy_doMenor8/1 -> Gateway Out37/1, Sum_wxWinning_n7/2
  Gateway Out38/1 -> Display13/1
  Gateway Out39/1 -> Display14/1
  Gateway Out40/1 -> Display15/1
  Gateway Out41/1 -> Display16/1
  Gateway Out42/1 -> Display17/1
  Gateway Out43/1 -> Display18/1
  Gateway Out44/1 -> Display19/1
  Gateway Out45/1 -> Display20/1
  Gateway Out46/1 -> Display21/1
  Gateway Out47/1 -> Display22/1
  Gateway Out48/1 -> Display23/1
  Gateway Out49/1 -> Display24/1
  Gateway Out50/1 -> Display25/1
  Gateway Out51/1 -> Display26/1
  Gateway Out52/1 -> Display27/1
  wy_doMenor23/1 -> Gateway Out52/1, Sum_wxWinning_n21/2
  Gateway Out53/1 -> Display28/1
  Gateway Out54/1 -> Display29/1
  Gateway Out55/1 -> Display30/1
  Gateway Out56/1 -> Display31/1
  Gateway Out57/1 -> Display32/1
  Gateway Out58/1 -> Display33/1
  Gateway Out59/1 -> Display34/1
  Gateway Out60/1 -> Display35/1
  Gateway Out61/1 -> Display36/1
  Gateway Out62/1 -> Display37/1
  Gateway Out63/1 -> Display38/1
  Gateway Out64/1 -> Display39/1
  Gateway Out65/1 -> Display40/1
  Gateway Out66/1 -> Display41/1
  Gateway Out67/1 -> Display42/1
  Gateway Out68/1 -> Display43/1
  Gateway Out69/1 -> Display44/1
  Gateway Out70/1 -> Display45/1
  Gateway Out71/1 -> Display46/1
  Gateway Out72/1 -> Display47/1
  Gateway Out73/1 -> Display48/1
  Gateway Out74/1 -> Display49/1
  wy_doMenor45/1 -> Gateway Out74/1, Sum_wxWinning_n43/2
  Gateway Out75/1 -> Display50/1
  Gateway Out76/1 -> Display51/1
  Gateway Out77/1 -> Display52/1
  Gateway Out78/1 -> Display53/1
  dist_k5/1 -> LowerDist_n1/5(In5), LowerDist_n25/5(In5), LowerDist_n24/5(In5), LowerDist_n23/5(In5), LowerDist_n22/5(In5), LowerDist_n21/5(In5), LowerDist_n20/5(In5), LowerDist_n19/5(In5), LowerDist_n18/5(In5), LowerDist_n17/5(In5), LowerDist_n16/5(In5), LowerDist_n15/5(In5), LowerDist_n14/5(In5), LowerDist_n13/5(In5), LowerDist_n12/5(In5), LowerDist_n11/5(In5), LowerDist_n10/5(In5), LowerDist_n9/5(In5), LowerDist_n8/5(In5), LowerDist_n7/5(In5), LowerDist_n6/5(In5), LowerDist_n5/1(In1), LowerDist_n4/5(In5), LowerDist_n3/5(In5), LowerDist_n2/5(In5), Gateway Out4/1
  Mux/1 -> Minimum/1, Display1/1, Sort/1
  Minimum/2 -> Display/1
  Minimum/1 -> Display2/1, To Workspace1/1
  Sort/1 -> Display54/1
  Sort/2 -> Display55/1, To Workspace/1
  LowerDist_n2/1(Out1) -> wy_doMenor50/2
  zero50/1 -> wy_doMenor50/3
  wy_doMenor50/1 -> wy_doMenor2/1, wy_doMenor3/1, Logical/2
  LowerDist_n1/1(Out1) -> wy_doMenor/1, Logical/1, wy_doMenor50/1, wy_doMenor1/1
  LowerDist_n3/1(Out1) -> wy_doMenor51/2
  wy_doMenor51/1 -> wy_doMenor4/1, Logical1/2, wy_doMenor5/1
  Logical/1 -> wy_doMenor51/1, Logical1/1
  LowerDist_n4/1(Out1) -> wy_doMenor52/2
  wy_doMenor52/1 -> wy_doMenor6/1, Logical2/2, wy_doMenor7/1
  Logical1/1 -> wy_doMenor52/1, Logical2/1
  LowerDist_n5/1(Out1) -> wy_doMenor53/2
  wy_doMenor53/1 -> wy_doMenor8/1, wy_doMenor9/1, Logical3/2
  Logical2/1 -> wy_doMenor53/1, Logical3/1
  LowerDist_n6/1(Out1) -> wy_doMenor54/2
  wy_doMenor54/1 -> wy_doMenor10/1, Logical4/2, wy_doMenor11/1
  Logical3/1 -> wy_doMenor54/1, Logical4/1
  LowerDist_n7/1(Out1) -> wy_doMenor55/2
  wy_doMenor55/1 -> wy_doMenor12/1, Logical5/2, wy_doMenor13/1
  Logical4/1 -> wy_doMenor55/1, Logical5/1
  LowerDist_n8/1(Out1) -> wy_doMenor56/2
  wy_doMenor56/1 -> wy_doMenor14/1, Logical6/2, wy_doMenor15/1
  Logical5/1 -> wy_doMenor56/1, Logical6/1
  LowerDist_n9/1(Out1) -> wy_doMenor57/2
  wy_doMenor57/1 -> wy_doMenor16/1, Logical7/2, wy_doMenor17/1
  Logical6/1 -> wy_doMenor57/1, Logical7/1
  LowerDist_n10/1(Out1) -> wy_doMenor58/2
  wy_doMenor58/1 -> wy_doMenor18/1, Logical8/2, wy_doMenor19/1
  Logical7/1 -> wy_doMenor58/1, Logical8/1
  LowerDist_n11/1(Out1) -> wy_doMenor59/2
  wy_doMenor59/1 -> wy_doMenor20/1, Logical9/2, wy_doMenor21/1
  Logical8/1 -> wy_doMenor59/1, Logical9/1
  LowerDist_n12/1(Out1) -> wy_doMenor60/2
  wy_doMenor60/1 -> wy_doMenor22/1, wy_doMenor23/1, Logical10/2
  Logical9/1 -> wy_doMenor60/1, Logical10/1
  LowerDist_n13/1(Out1) -> wy_doMenor61/2
  wy_doMenor61/1 -> wy_doMenor24/1, Logical11/2, wy_doMenor25/1
  Logical10/1 -> wy_doMenor61/1, Logical11/1
  LowerDist_n14/1(Out1) -> wy_doMenor62/2
  wy_doMenor62/1 -> wy_doMenor26/1, wy_doMenor27/1, Logical12/2
  Logical11/1 -> wy_doMenor62/1, Logical12/1
  LowerDist_n15/1(Out1) -> wy_doMenor63/2
  wy_doMenor63/1 -> wy_doMenor28/1, Logical13/2, wy_doMenor29/1
  Logical12/1 -> wy_doMenor63/1, Logical13/1
  LowerDist_n16/1(Out1) -> wy_doMenor64/2
  wy_doMenor64/1 -> wy_doMenor30/1, wy_doMenor31/1, Logical14/2
  Logical13/1 -> wy_doMenor64/1, Logical14/1
  LowerDist_n17/1(Out1) -> wy_doMenor65/2
  wy_doMenor65/1 -> wy_doMenor32/1, Logical15/2, wy_doMenor33/1
  Logical14/1 -> wy_doMenor65/1, Logical15/1
  LowerDist_n18/1(Out1) -> wy_doMenor66/2
  wy_doMenor66/1 -> wy_doMenor34/1, Logical16/2, wy_doMenor35/1
  Logical15/1 -> wy_doMenor66/1, Logical16/1
  LowerDist_n19/1(Out1) -> wy_doMenor67/2
  wy_doMenor67/1 -> wy_doMenor36/1, wy_doMenor37/1, Logical17/2
  Logical16/1 -> wy_doMenor67/1, Logical17/1
  LowerDist_n20/1(Out1) -> wy_doMenor68/2
  wy_doMenor68/1 -> wy_doMenor38/1, Logical18/2, wy_doMenor39/1
  Logical17/1 -> wy_doMenor68/1, Logical18/1
  LowerDist_n21/1(Out1) -> wy_doMenor69/2
  wy_doMenor69/1 -> wy_doMenor40/1, Logical19/2, wy_doMenor41/1
  Logical18/1 -> wy_doMenor69/1, Logical19/1
  LowerDist_n22/1(Out1) -> wy_doMenor70/2
  wy_doMenor70/1 -> wy_doMenor42/1, Logical20/2, wy_doMenor43/1
  Logical19/1 -> wy_doMenor70/1, Logical20/1
  LowerDist_n23/1(Out1) -> wy_doMenor71/2
  wy_doMenor71/1 -> wy_doMenor44/1, Logical21/2, wy_doMenor45/1
  Logical20/1 -> wy_doMenor71/1, Logical21/1
  LowerDist_n24/1(Out1) -> wy_doMenor72/2
  wy_doMenor72/1 -> wy_doMenor46/1, Logical22/2, wy_doMenor47/1
  Logical21/1 -> wy_doMenor72/1, Logical22/1
  LowerDist_n25/1(Out1) -> wy_doMenor73/2
  wy_doMenor73/1 -> wy_doMenor48/1, wy_doMenor49/1
  Logical22/1 -> wy_doMenor73/1
  zero51/1 -> wy_doMenor51/3
  zero52/1 -> wy_doMenor52/3
  zero53/1 -> wy_doMenor53/3
  zero54/1 -> wy_doMenor54/3
  zero55/1 -> wy_doMenor55/3
  zero56/1 -> wy_doMenor56/3
  zero57/1 -> wy_doMenor57/3
  zero58/1 -> wy_doMenor58/3
  zero59/1 -> wy_doMenor59/3
  zero60/1 -> wy_doMenor60/3
  zero61/1 -> wy_doMenor61/3
  zero62/1 -> wy_doMenor62/3
  zero63/1 -> wy_doMenor63/3
  zero64/1 -> wy_doMenor64/3
  zero65/1 -> wy_doMenor65/3
  zero66/1 -> wy_doMenor66/3
  zero67/1 -> wy_doMenor67/3
  zero68/1 -> wy_doMenor68/3
  zero69/1 -> wy_doMenor69/3
  zero70/1 -> wy_doMenor70/3
  zero71/1 -> wy_doMenor71/3
  zero72/1 -> wy_doMenor72/3
  zero73/1 -> wy_doMenor73/3

== system Parallel_n25_D2/Neurons/Neuron1 ==
  note: Checking difference between input data and neuron weight
  note: 1. Obtain the distance between this neuron and and winning neuron coordinates
      | 2. Obtaining neighborhood distance: h=exp(-1*(dist²/2S²))
  note: Cooperating Process
  note: Adaptive Process
  note: Updating weights: w(n+1)=wn+N*h*dif
  vX11 : Inport
  vX12 : Inport  Port=2
  S : Inport  Port=3
  N : Inport  Port=4
  MemoryControl : Inport  Port=5
  wx_n1 : Inport  Port=6
  wy_n1 : Inport  Port=7
  wxWinningNeuron : Inport  Port=8
  wyWinningNeuron : Inport  Port=9
  Absolute{,1..3} (4 alike) : xbsIndex_r4/Absolute  precision=Full  arith_type=Unsigned  n_bits=16  bin_pt=14  quantization=Truncate  overflow=Wrap  en=off  latency=dSub_CompetitiveProcess  dbl_ovrd=off  block_type=abs
  CMult : xbsIndex_r4/CMult  const=(2^nBits)/MaxCoordDistance  gui_display_data_type=Fixed-point  const_n_bits=nbGainBlock  const_bin_pt=bpSNMemory  float_type=Single  exp_bits=8  fraction_bits=24  en=off  latency=dGain_CooperatingProcess  precision=User Defined  arith_type=Unsigned  n_bits=nBits  bin_pt=0  quantization="Round  (unbiased: +/- Inf)"  overflow=Wrap  dbl_ovrd=off  use_behavioral_HDL=off  mem_type=Block RAM  pipeline=off  block_type=cmult
  Delay_vX11 : xbsIndex_r4/Delay  rst=off  infoeditControl=Selection of Reset will increase slice count due to use of real FFs and instead of SRLs  en=off  latency=dDelay_CooperatingProcess  dbl_ovrd=off  reg_retiming=off  block_type=delay
  Delay_vX12 : xbsIndex_r4/Delay  rst=off  infoeditControl=Selection of Reset will increase slice count due to use of real FFs and instead of SRLs  en=off  latency=dDelay_CooperatingProcess  dbl_ovrd=off  reg_retiming=off  block_type=delay
  N*h*dif_w1n1 : xbsIndex_r4/Mult  precision=User Defined  arith_type="Signed  (2's comp)"  n_bits=nbMult  bin_pt=bpMult  quantization="Round  (unbiased: +/- Inf)"  overflow=Saturate  en=off  latency=dMult_CooperatingProcess  dbl_ovrd=off  use_behavioral_HDL=off  opt=Speed  use_embedded=on  optimum_pipeline=off  pipeline=on  use_rpm=on  placement_style=Triangular  block_type=mult
  N*h*dif_w2n1 : xbsIndex_r4/Mult  precision=User Defined  arith_type="Signed  (2's comp)"  n_bits=nbMult  bin_pt=bpMult  quantization="Round  (unbiased: +/- Inf)"  overflow=Saturate  en=off  latency=dMult_CooperatingProcess  dbl_ovrd=off  use_behavioral_HDL=off  opt=Speed  use_embedded=on  optimum_pipeline=off  pipeline=on  use_rpm=on  placement_style=Triangular  block_type=mult
  NeighboordFunction_H_n1 : xbsIndex_r4/ROM  depth=2^nBits  initVector=h  distributed_mem=Block RAM  rst=off  init_reg=0  en=on  latency=dMemoryNeighborFunc  gui_display_data_type=Fixed-point  arith_type=Unsigned  n_bits=bp+1  bin_pt=bp  preci_type=Single  exp_width=8  frac_width=24  dbl_ovrd=off  optimize=Area  use_rpm=on  block_type=sprom
  Sum_wxWinning_n1 : xbsIndex_r4/AddSub  mode=Addition  use_carryin=off  use_carryout=off  en=off  latency=dAdd_CooperatingProcess  precision=Full  arith_type=Unsigned  n_bits=nbCoord  bin_pt=bpCoord  quantization=Truncate  overflow=Wrap  dbl_ovrd=off  use_behavioral_HDL=off  hw_selection=Fabric  pipelined=off  block_type=addsub
  Sum_x1n1 : xbsIndex_r4/AddSub  mode=Addition  use_carryin=off  use_carryout=off  en=off  latency=dAdd_CompetitiveProcess  precision=Full  arith_type=Unsigned  n_bits=nb  bin_pt=bp  quantization=Truncate  overflow=Wrap  dbl_ovrd=off  use_behavioral_HDL=off  hw_selection=Fabric  pipelined=off  block_type=addsub
  h*dif_w1n1 : xbsIndex_r4/Mult  precision=User Defined  arith_type="Signed  (2's comp)"  n_bits=nbMult  bin_pt=bpMult  quantization="Round  (unbiased: +/- Inf)"  overflow=Saturate  en=off  latency=dMult_CooperatingProcess  dbl_ovrd=off  use_behavioral_HDL=off  opt=Speed  use_embedded=on  optimum_pipeline=off  pipeline=on  use_rpm=on  placement_style=Triangular  block_type=mult
  h*dif_w1n2 : xbsIndex_r4/Mult  precision=User Defined  arith_type=Unsigned  n_bits=nbCoordMult  bin_pt=bpCoordMult  quantization="Round  (unbiased: +/- Inf)"  overflow=Saturate  en=off  latency=dMult_CooperatingProcess  dbl_ovrd=off  use_behavioral_HDL=off  opt=Speed  use_embedded=on  optimum_pipeline=off  pipeline=on  use_rpm=on  placement_style=Triangular  block_type=mult
  h*dif_w2n1 : xbsIndex_r4/Mult  precision=User Defined  arith_type="Signed  (2's comp)"  n_bits=nbMult  bin_pt=bpMult  quantization="Round  (unbiased: +/- Inf)"  overflow=Saturate  en=off  latency=dMult_CooperatingProcess  dbl_ovrd=off  use_behavioral_HDL=off  opt=Speed  use_embedded=on  optimum_pipeline=off  pipeline=on  use_rpm=on  placement_style=Triangular  block_type=mult
  h_adress1 : xbsIndex_r4/Mult  precision=User Defined  arith_type=Unsigned  n_bits=nb  bin_pt=bp  quantization="Round  (unbiased: +/- Inf)"  overflow=Saturate  en=off  latency=dMultAddress_CooperatingProcess  dbl_ovrd=off  use_behavioral_HDL=off  opt=Speed  use_embedded=on  optimum_pipeline=off  pipeline=on  use_rpm=on  placement_style=Triangular  block_type=mult
  vX12_n1 : xbsIndex_r4/AddSub  mode=Subtraction  use_carryin=off  use_carryout=off  en=off  latency=dSub_CompetitiveProcess  precision=User Defined  arith_type="Signed  (2's comp)"  n_bits=nb  bin_pt=bp  quantization=Truncate  overflow=Wrap  dbl_ovrd=off  use_behavioral_HDL=off  hw_selection=Fabric  pipelined=on  block_type=addsub
  w1n1 : xbsIndex_r4/Register  init=w1(1)  rst=off  en=off  dbl_ovrd=off  block_type=register
  w2n1 : xbsIndex_r4/Register  init=w2(1)  rst=off  en=off  dbl_ovrd=off  block_type=register
  wx+N*h*dif_w1n1 : xbsIndex_r4/AddSub  mode=Addition  use_carryin=off  use_carryout=off  en=off  latency=dSub_CooperatingProcess  precision=User Defined  arith_type="Signed  (2's comp)"  n_bits=nb  bin_pt=bp  quantization=Truncate  overflow=Wrap  dbl_ovrd=off  use_behavioral_HDL=off  hw_selection=Fabric  pipelined=off  block_type=addsub
  wx+N*h*dif_w2n1 : xbsIndex_r4/AddSub  mode=Addition  use_carryin=off  use_carryout=off  en=off  latency=dSub_CooperatingProcess  precision=User Defined  arith_type="Signed  (2's comp)"  n_bits=nb  bin_pt=bp  quantization=Truncate  overflow=Wrap  dbl_ovrd=off  use_behavioral_HDL=off  hw_selection=Fabric  pipelined=off  block_type=addsub
  wy_wyWinning_n1 : xbsIndex_r4/AddSub  mode=Subtraction  use_carryin=off  use_carryout=off  en=off  latency=dSub_CooperatingProcess  precision=User Defined  arith_type="Signed  (2's comp)"  n_bits=nbCoord  bin_pt=bpCoord  quantization=Truncate  overflow=Wrap  dbl_ovrd=off  use_behavioral_HDL=off  hw_selection=Fabric  pipelined=on  block_type=addsub
  wy_wyWinning_n2 : xbsIndex_r4/AddSub  mode=Subtraction  use_carryin=off  use_carryout=off  en=off  latency=dSub_CooperatingProcess  precision=User Defined  arith_type="Signed  (2's comp)"  n_bits=nbCoord  bin_pt=bpCoord  quantization=Truncate  overflow=Wrap  dbl_ovrd=off  use_behavioral_HDL=off  hw_selection=Fabric  pipelined=on  block_type=addsub
  x11_n1 : xbsIndex_r4/AddSub  mode=Subtraction  use_carryin=off  use_carryout=off  en=off  latency=dSub_CompetitiveProcess  precision=User Defined  arith_type="Signed  (2's comp)"  n_bits=nb  bin_pt=bp  quantization=Truncate  overflow=Wrap  dbl_ovrd=off  use_behavioral_HDL=off  hw_selection=Fabric  pipelined=on  block_type=addsub
  w1-n1 : Outport
  w2-n1 : Outport  Port=2
  dist_n1 : Outport  Port=3
  wires:
  wy_wyWinning_n1/1 -> Absolute3/1
  Absolute3/1 -> Sum_wxWinning_n1/2
  Absolute2/1 -> Sum_wxWinning_n1/1
  wy_wyWinning_n2/1 -> Absolute2/1
  h_adress1/1 -> CMult/1
  CMult/1 -> NeighboordFunction_H_n1/1
  S/1 -> h_adress1/1
  wxWinningNeuron/1 -> wy_wyWinning_n2/2
  wy_n1/1 -> wy_wyWinning_n1/1
  wyWinningNeuron/1 -> wy_wyWinning_n1/2
  MemoryControl/1 -> NeighboordFunction_H_n1/2
  h*dif_w2n1/1 -> N*h*dif_w2n1/2
  h*dif_w1n1/1 -> N*h*dif_w1n1/2
  N*h*dif_w2n1/1 -> wx+N*h*dif_w2n1/1
  N*h*dif_w1n1/1 -> wx+N*h*dif_w1n1/2
  wx+N*h*dif_w1n1/1 -> w1n1/1, x11_n1/2
  w1n1/1 -> w1-n1/1, wx+N*h*dif_w1n1/1
  wx+N*h*dif_w2n1/1 -> vX12_n1/2, w2n1/1
  w2n1/1 -> w2-n1/1, wx+N*h*dif_w2n1/2
  NeighboordFunction_H_n1/1 -> h*dif_w2n1/1, h*dif_w1n1/1
  x11_n1/1 -> Delay_vX11/1, Absolute/1
  vX12_n1/1 -> Delay_vX12/1, Absolute1/1
  Absolute/1 -> Sum_x1n1/1
  Absolute1/1 -> Sum_x1n1/2
  vX12/1 -> vX12_n1/1
  vX11/1 -> x11_n1/1
  Sum_x1n1/1 -> dist_n1/1
  Delay_vX11/1 -> h*dif_w1n1/2
  Delay_vX12/1 -> h*dif_w2n1/2
  h*dif_w1n2/1 -> h_adress1/2
  Sum_wxWinning_n1/1 -> h*dif_w1n2/2, h*dif_w1n2/1
  N/1 -> N*h*dif_w2n1/1, N*h*dif_w1n1/1
  wx_n1/1 -> wy_wyWinning_n2/1
